simulink model "Lab4"  (R2012b)
settings: Solver=ode45  StartTime=0.0  StopTime=500  RelTol=1e-3
settings Model: Creator=Viktor  LastModifiedBy=Viktor

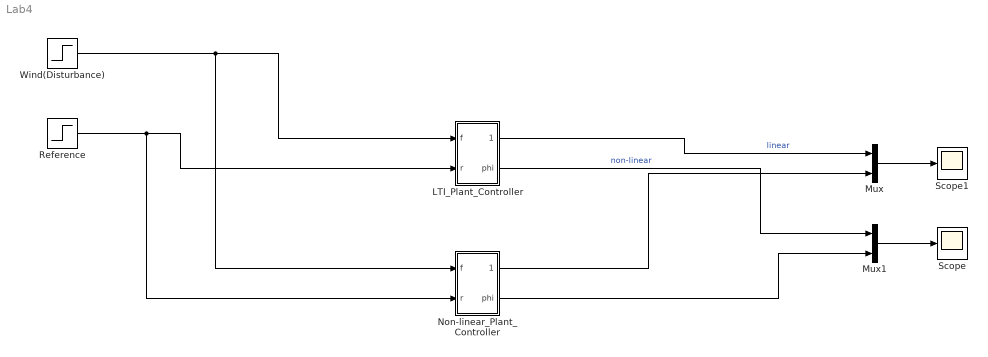
== system Lab4 ==
  LTI_Plant_Controller : Subsystem
  Mux : Mux  Inputs=2
  Mux1 : Mux  Inputs=2
  Non-linear_Plant_Controller : Subsystem
  Reference : Step  Time=0  After=10  SampleTime=0
  Scope : Scope
  Scope1 : Scope
  Wind(Disturbance) : Step  Time=0  After=2  SampleTime=0
  wires:
  Wind(Disturbance)/1 -> Non-linear_Plant_Controller/1(f), LTI_Plant_Controller/1(f)
  Reference/1 -> Non-linear_Plant_Controller/2(r), LTI_Plant_Controller/2(r)
  LTI_Plant_Controller/1(delta) -> Mux/1  "linear"
  Mux/1 -> Scope1/1
  Non-linear_Plant_Controller/2(phi) -> Mux1/2
  Mux1/1 -> Scope/1
  Non-linear_Plant_Controller/1(delta) -> Mux/2
  LTI_Plant_Controller/2(phi) -> Mux1/1  "non-linear"

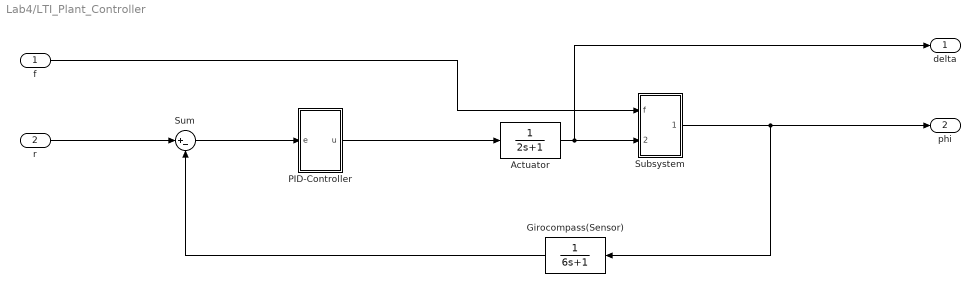
== system Lab4/LTI_Plant_Controller ==
  f : Inport
  r : Inport  Port=2
  Actuator : TransferFcn  Denominator=[2 1]
  Girocompass(Sensor) : TransferFcn  Denominator=[6 1]
  PID-Controller : Subsystem
  Subsystem : Subsystem
  Sum : Sum  Inputs=|+-
  delta : Outport
  phi : Outport  Port=2
  wires:
  r/1 -> Sum/1
  Girocompass(Sensor)/1 -> Sum/2
  Sum/1 -> PID-Controller/1(e)
  PID-Controller/1(u) -> Actuator/1
  Actuator/1 -> delta/1, Subsystem/2(delta)
  f/1 -> Subsystem/1("f ")
  Subsystem/1(phi) -> phi/1, Girocompass(Sensor)/1

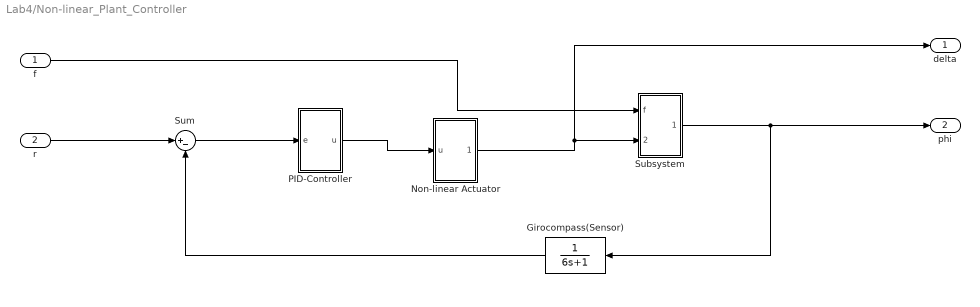
== system Lab4/Non-linear_Plant_Controller ==
  f : Inport
  r : Inport  Port=2
  Girocompass(Sensor) : TransferFcn  Denominator=[6 1]
  Non-linear Actuator : Subsystem
  PID-Controller : Subsystem
  Subsystem : Subsystem
  Sum : Sum  Inputs=|+-
  delta : Outport
  phi : Outport  Port=2
  wires:
  Subsystem/1(phi) -> Girocompass(Sensor)/1, phi/1
  f/1 -> Subsystem/1("f ")
  Sum/1 -> PID-Controller/1(e)
  Girocompass(Sensor)/1 -> Sum/2
  r/1 -> Sum/1
  Non-linear Actuator/1(delta) -> Subsystem/2(delta), delta/1
  PID-Controller/1(u) -> Non-linear Actuator/1(u)

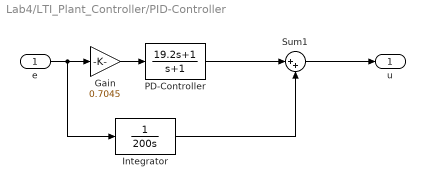
== system Lab4/LTI_Plant_Controller/PID-Controller ==
  e : Inport
  Gain : Gain  Gain=0.7045
  Integrator : TransferFcn  Denominator=[200 0]
  PD-Controller : TransferFcn  Numerator=[19.2 1]  Denominator=[1 1]
  Sum1 : Sum  Inputs=|++
  u : Outport
  wires:
  Sum1/1 -> u/1
  Gain/1 -> PD-Controller/1
  e/1 -> Integrator/1, Gain/1
  PD-Controller/1 -> Sum1/1
  Integrator/1 -> Sum1/2

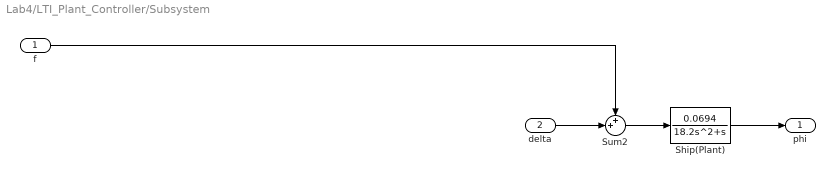
== system Lab4/LTI_Plant_Controller/Subsystem ==
  "f " : Inport
  delta : Inport  Port=2
  Ship(Plant) : TransferFcn  Numerator=[0.0694]  Denominator=[18.2 1 0]
  Sum2 : Sum  Inputs=++|
  phi : Outport
  wires:
  Ship(Plant)/1 -> phi/1
  Sum2/1 -> Ship(Plant)/1
  "f "/1 -> Sum2/1
  delta/1 -> Sum2/2

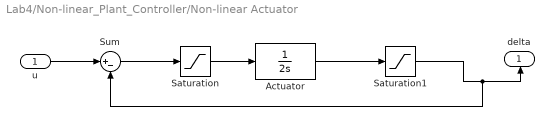
== system Lab4/Non-linear_Plant_Controller/Non-linear Actuator ==
  u : Inport
  Actuator : TransferFcn  Denominator=[2 0]
  Saturation : Saturate  UpperLimit=3  LowerLimit=-3
  Saturation1 : Saturate  UpperLimit=30  LowerLimit=-30
  Sum : Sum  Inputs=|+-
  delta : Outport
  wires:
  u/1 -> Sum/1
  Sum/1 -> Saturation/1
  Saturation/1 -> Actuator/1
  Actuator/1 -> Saturation1/1
  Saturation1/1 -> Sum/2, delta/1

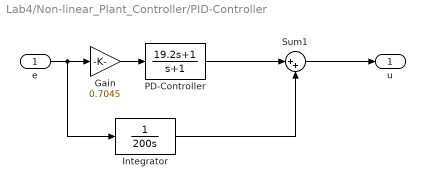
== system Lab4/Non-linear_Plant_Controller/PID-Controller ==
  e : Inport
  Gain : Gain  Gain=0.7045
  Integrator : TransferFcn  Denominator=[200 0]
  PD-Controller : TransferFcn  Numerator=[19.2 1]  Denominator=[1 1]
  Sum1 : Sum  Inputs=|++
  u : Outport
  wires:
  Integrator/1 -> Sum1/2
  PD-Controller/1 -> Sum1/1
  e/1 -> Gain/1, Integrator/1
  Gain/1 -> PD-Controller/1
  Sum1/1 -> u/1

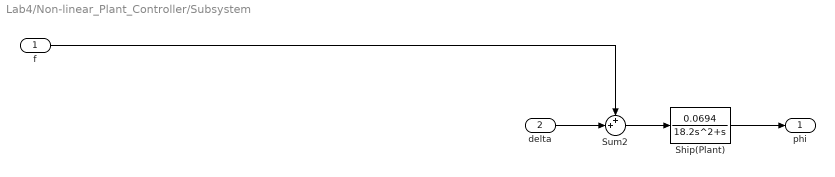
== system Lab4/Non-linear_Plant_Controller/Subsystem ==
  "f " : Inport
  delta : Inport  Port=2
  Ship(Plant) : TransferFcn  Numerator=[0.0694]  Denominator=[18.2 1 0]
  Sum2 : Sum  Inputs=++|
  phi : Outport
  wires:
  delta/1 -> Sum2/2
  "f "/1 -> Sum2/1
  Sum2/1 -> Ship(Plant)/1
  Ship(Plant)/1 -> phi/1
